simulink model "Washingmachine"  (R2024b)
settings: Solver=VariableStepAuto  StartTime=0.0  StopTime=inf  RelTol=1e-3
settings Model: Creator=HP  LastModifiedBy=HP

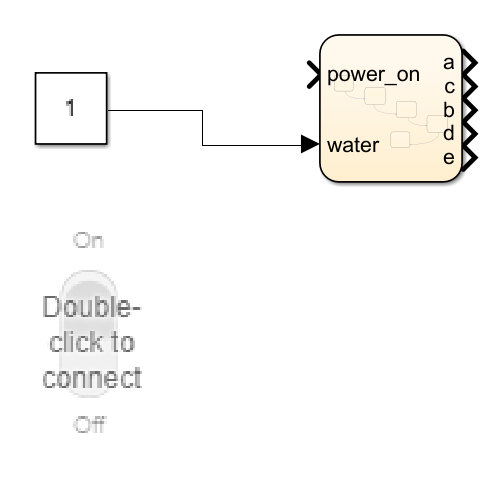
[thumbnail: Simulink's stored preview of the top-level diagram]
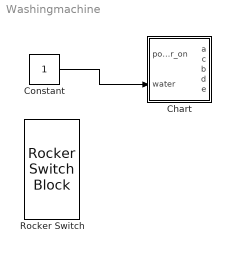
== system Washingmachine ==
  Chart : Stateflow chart  TreatAsAtomicUnit=on
  Constant : Constant
  Rocker Switch : RockerSwitchBlock
      settings: Values={{'Off', 'On'}, [0 1]}
  wires:
  Constant/1 -> Chart/2(water)

== stateflow chart Washingmachine/Chart ==
  state fill
    entry:
    a=1;
  state wash
    entry:
    a=0;
    during:
    b=1;
  state rinse
    entry:
    b=0;
    during:
    c=1;
  state spin
    entry:
    c=0;
    during:
    d=1;
  state done
    entry:
    d=0;
    during:
    e=1;
  (default) -> fill : {power_on==1}
  fill -> wash : [water==1]
  wash -> rinse : after(40,sec)
  rinse -> spin : after(20,sec)
  spin -> done : after(20,sec)
  data: power_on input; water input; a output; c output; b output; d output; e output
